simulink model "laboratorium"  (Simulink 7.5)
settings: Solver=ode45  StartTime=0.0  StopTime=20  RelTol=1e-3
undefined symbols (not defined in the file): b, c, Kr, ogr, Td, Tdf, Ti, Tp, Tt, yref
settings Model: Creator=sieklo  LastModifiedBy=Konrad

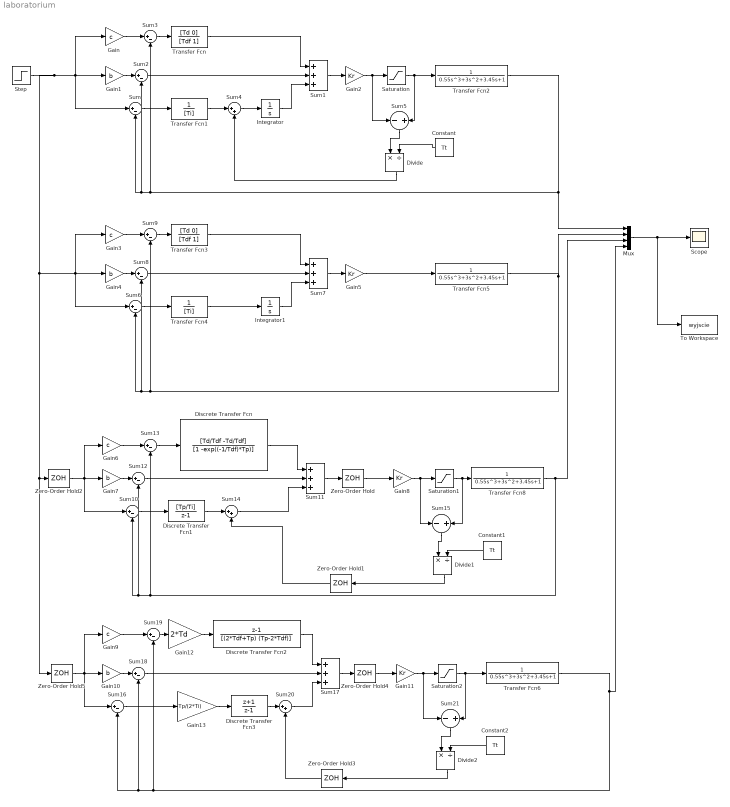
== system laboratorium ==
  Constant : Constant  Value=Tt
  Constant1 : Constant  Value=Tt
  Constant2 : Constant  Value=Tt
  Discrete Transfer Fcn : DiscreteTransferFcn  Numerator=[Td/Tdf -Td/Tdf]  Denominator=[1 -exp((-1/Tdf)*Tp)]  SampleTime=Tp
  Discrete Transfer Fcn1 : DiscreteTransferFcn  Numerator=[Tp/Ti]  Denominator=[1 -1]  SampleTime=Tp
  Discrete Transfer Fcn2 : DiscreteTransferFcn  Numerator=[1 -1]  Denominator=[(2*Tdf+Tp) (Tp-2*Tdf)]  SampleTime=Tp
  Discrete Transfer Fcn3 : DiscreteTransferFcn  Numerator=[1 1]  Denominator=[1 -1]  SampleTime=Tp
  Divide : Product  Inputs=*/
  Divide1 : Product  Inputs=*/
  Divide2 : Product  Inputs=*/
  Gain{,3,6,9} (4 alike) : Gain  Gain=c
  Gain{1,4,7,10} (4 alike) : Gain  Gain=b
  Gain{2,5,8,11} (4 alike) : Gain  Gain=Kr
  Gain12 : Gain  Gain=2*Td  ParameterDataType=fixdt(1, 16)  ParameterScaling=2^0  OutDataType=fixdt(1, 16)  OutScaling=2^0
  Gain13 : Gain  Gain=Tp/(2*Ti)
  Integrator : Integrator  LimitOutput=on  UpperSaturationLimit=1  LowerSaturationLimit=-1
  Integrator1 : Integrator  LimitOutput=on  UpperSaturationLimit=1  LowerSaturationLimit=-1
  Mux : Mux
  Saturation : Saturate  UpperLimit=ogr  LowerLimit=-ogr
  Saturation1 : Saturate  UpperLimit=ogr  LowerLimit=-ogr
  Saturation2 : Saturate  UpperLimit=ogr  LowerLimit=-ogr
  Scope : Scope
  Step : Step  Time=0  After=yref  SampleTime=0
  Sum{,2..3,6,8..10,12..13,16,18..19} (12 alike) : Sum  Inputs=|+-
  Sum{1,7,11,17} (4 alike) : Sum  Inputs=+++
  Sum14 : Sum  Inputs=|++
  Sum15 : Sum  Inputs=-+
  Sum20 : Sum  Inputs=|++
  Sum21 : Sum  Inputs=-+
  Sum4 : Sum  Inputs=|++
  Sum5 : Sum  Inputs=-+
  To Workspace : ToWorkspace  VariableName=wyjscie  SampleTime=-1  SaveFormat=Structure
  Transfer Fcn : TransferFcn  Numerator=[Td 0]  Denominator=[Tdf 1]
  Transfer Fcn1 : TransferFcn  Denominator=[Ti]
  Transfer Fcn{2,5..6,8} (4 alike) : TransferFcn  Denominator=[0.55 3 3.45 1]
  Transfer Fcn3 : TransferFcn  Numerator=[Td 0]  Denominator=[Tdf 1]
  Transfer Fcn4 : TransferFcn  Denominator=[Ti]
  Zero-Order Hold{,1..5} (6 alike) : ZeroOrderHold  SampleTime=Tp
  wires:
  Sum/1 -> Transfer Fcn1/1
  Transfer Fcn/1 -> Sum1/1
  Sum3/1 -> Transfer Fcn/1
  Gain/1 -> Sum3/1
  Step/1 -> Gain1/1, Gain/1, Sum/1, Gain4/1, Gain3/1, Sum6/1, Zero-Order Hold2/1, Zero-Order Hold5/1
  Gain1/1 -> Sum2/1
  Sum2/1 -> Sum1/2
  Sum4/1 -> Integrator/1
  Transfer Fcn1/1 -> Sum4/1
  Integrator/1 -> Sum1/3
  Saturation/1 -> Sum5/2, Transfer Fcn2/1
  Gain2/1 -> Saturation/1, Sum5/1
  Sum1/1 -> Gain2/1
  Transfer Fcn2/1 -> Sum/2, Sum2/2, Sum3/2, Mux/1
  Divide/1 -> Sum4/2
  Sum5/1 -> Divide/1
  Constant/1 -> Divide/2
  Sum6/1 -> Transfer Fcn4/1
  Transfer Fcn3/1 -> Sum7/1
  Sum9/1 -> Transfer Fcn3/1
  Gain3/1 -> Sum9/1
  Gain4/1 -> Sum8/1
  Sum8/1 -> Sum7/2
  Transfer Fcn4/1 -> Integrator1/1
  Integrator1/1 -> Sum7/3
  Gain5/1 -> Transfer Fcn5/1
  Sum7/1 -> Gain5/1
  Transfer Fcn5/1 -> Sum6/2, Sum8/2, Sum9/2, Mux/2
  Mux/1 -> Scope/1, To Workspace/1
  Sum10/1 -> Discrete Transfer Fcn1/1
  Discrete Transfer Fcn/1 -> Sum11/1
  Sum13/1 -> Discrete Transfer Fcn/1
  Gain6/1 -> Sum13/1
  Gain7/1 -> Sum12/1
  Sum12/1 -> Sum11/2
  Sum14/1 -> Sum11/3
  Discrete Transfer Fcn1/1 -> Sum14/1
  Saturation1/1 -> Sum15/2, Transfer Fcn8/1
  Gain8/1 -> Saturation1/1, Sum15/1
  Sum11/1 -> Zero-Order Hold/1
  Transfer Fcn8/1 -> Sum10/2, Sum12/2, Sum13/2, Mux/3
  Divide1/1 -> Zero-Order Hold1/1
  Sum15/1 -> Divide1/1
  Constant1/1 -> Divide1/2
  Sum16/1 -> Gain13/1
  Discrete Transfer Fcn2/1 -> Sum17/1
  Gain9/1 -> Sum19/1
  Gain10/1 -> Sum18/1
  Sum18/1 -> Sum17/2
  Sum20/1 -> Sum17/3
  Discrete Transfer Fcn3/1 -> Sum20/1
  Saturation2/1 -> Sum21/2, Transfer Fcn6/1
  Gain11/1 -> Saturation2/1, Sum21/1
  Sum17/1 -> Zero-Order Hold4/1
  Transfer Fcn6/1 -> Sum16/2, Sum18/2, Sum19/2, Mux/4
  Divide2/1 -> Zero-Order Hold3/1
  Sum21/1 -> Divide2/1
  Constant2/1 -> Divide2/2
  Gain12/1 -> Discrete Transfer Fcn2/1
  Sum19/1 -> Gain12/1
  Gain13/1 -> Discrete Transfer Fcn3/1
  Zero-Order Hold2/1 -> Gain7/1, Gain6/1, Sum10/1
  Zero-Order Hold/1 -> Gain8/1
  Zero-Order Hold1/1 -> Sum14/2
  Zero-Order Hold3/1 -> Sum20/2
  Zero-Order Hold4/1 -> Gain11/1
  Zero-Order Hold5/1 -> Gain10/1, Gain9/1, Sum16/1
